simulink model "controladoresDatosProyecto"  (R2022b)
settings: Solver=VariableStepAuto  StartTime=0.0  StopTime=1000  RelTol=1e-3
values from neighbouring files (symbols this model uses):
  kd = k4    (= 0.5686)    [controladoresDatosProyecto.m]
  ki = k1-kp1    (= 2.5726868)    [controladoresDatosProyecto.m]
  kp = k2-kd    (= 54.03607)    [controladoresDatosProyecto.m]
  kp1 = k2    (= 8.2233132)    [controladoresDatosProyecto.m]
  kp2 = k3-kd    (= 0.4314)    [controladoresDatosProyecto.m]
  N = 0.904    [controladoresDatosProyecto.m]
  Tm = 40e-3    (= 0.04)    [controladoresDatosProyecto.m]
undefined symbols (not defined in the file or in its folder): kaw, kpd, kpi
libraries: cstblocks x56
settings Model: Creator=Sebastian  LastModifiedBy=electronica
settings ModelReferenceCC: EnableRefExpFcnMdlSchedulingChecks=on

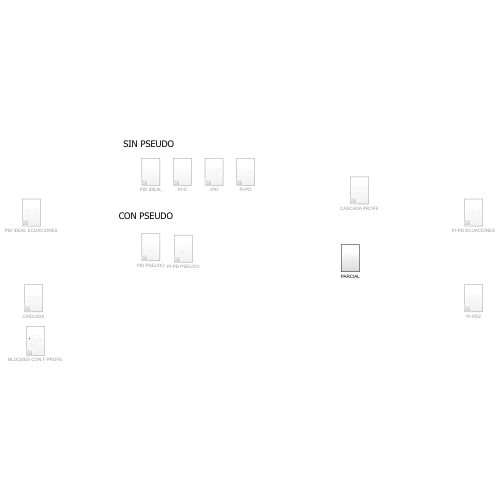
[thumbnail: Simulink's stored preview of the top-level diagram]
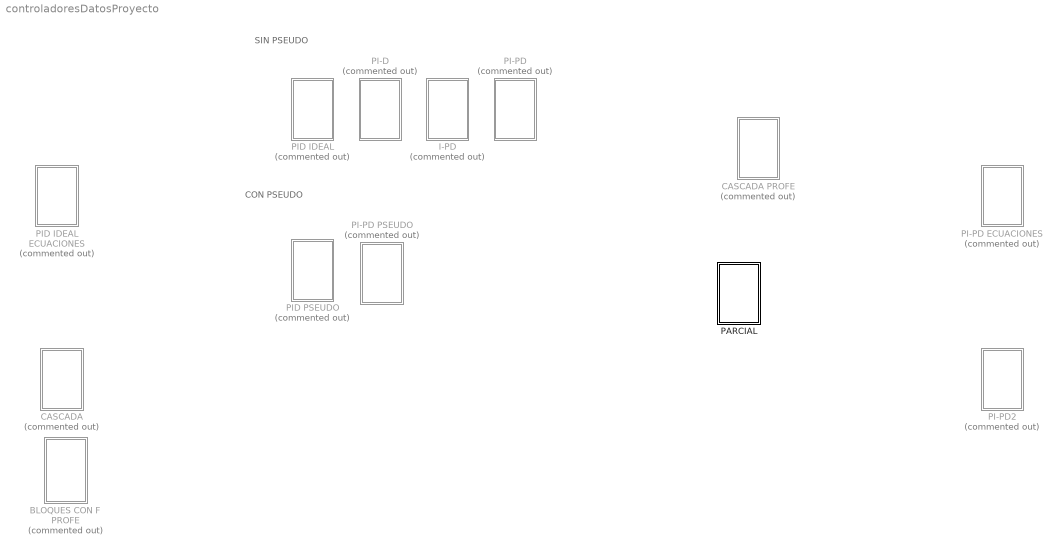
== system controladoresDatosProyecto ==
  note: SIN PSEUDO
  note: CON PSEUDO
  BLOQUES CON F PROFE : Subsystem  Commented=on
  CASCADA : Subsystem  Commented=on
  CASCADA PROFE : Subsystem  Commented=on
  I-PD : Subsystem  Commented=on
  PARCIAL : Subsystem
  PI-D : Subsystem  Commented=on
  PI-PD : Subsystem  Commented=on
  PI-PD ECUACIONES : Subsystem  Commented=on
  PI-PD PSEUDO : Subsystem  Commented=on
  PI-PD2 : Subsystem  Commented=on
  PID IDEAL : Subsystem  Commented=on
  PID IDEAL ECUACIONES : Subsystem  Commented=on
  PID PSEUDO : Subsystem  Commented=on

== system controladoresDatosProyecto/BLOQUES CON F PROFE ==
  LTI System : cstblocks/LTI System  sys=g  IC=[]
  LTI System1 : cstblocks/LTI System  sys=C  IC=[]
  LTI System2 : cstblocks/LTI System  sys=F  IC=[]
  LTI System3 : cstblocks/LTI System  sys=gz  IC=[]
  MATLAB Function : MATLAB Function  TreatAsAtomicUnit=on
  Mux : Mux  Inputs=3
  Mux1 : Mux  Inputs=2
  Scope : Scope  NumInputPorts=2
  Step : Step  Time=0  SampleTime=0
  Subtract : Sum
  Subtract1 : Sum  Inputs=+-
  Unit Delay : UnitDelay  InitialCondition=zeros(6,1)  SampleTime=0.2  HasFrameUpgradeWarning=on
  wires:
  LTI System1/1 -> Subtract/2
  LTI System/1 -> Subtract1/2, Mux/2
  Mux1/1 -> Scope/2
  MATLAB Function/2(Con_out) -> Unit Delay/1
  LTI System3/1 -> Mux/3, MATLAB Function/2(Pv)
  Unit Delay/1 -> MATLAB Function/3(Con_ini)
  Mux/1 -> Scope/1
  LTI System2/1 -> Subtract/1
  Step/1 -> Mux/1, LTI System2/1, MATLAB Function/1(Sp), Subtract1/1
  Subtract/1 -> LTI System/1, Mux1/1
  MATLAB Function/1(u) -> LTI System3/1, Mux1/2
  Subtract1/1 -> LTI System1/1

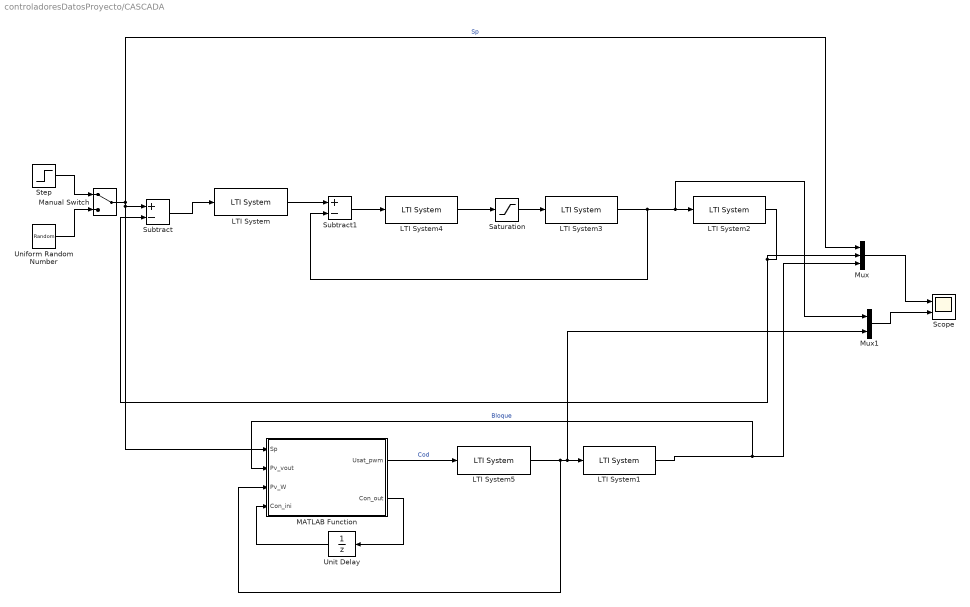
== system controladoresDatosProyecto/CASCADA ==
  LTI System : cstblocks/LTI System  sys=C1  IC=[]
  LTI System1 : cstblocks/LTI System  sys=G1z  IC=[]
  LTI System2 : cstblocks/LTI System  sys=G1z  IC=[]
  LTI System3 : cstblocks/LTI System  sys=G2z  IC=[]
  LTI System4 : cstblocks/LTI System  sys=C2  IC=[]
  LTI System5 : cstblocks/LTI System  sys=G2z  IC=[]
  MATLAB Function : MATLAB Function  TreatAsAtomicUnit=on
  Manual Switch : ManualSwitch
  Mux : Mux  Inputs=3
  Mux1 : Mux  Inputs=2
  Saturation : Saturate  UpperLimit=100  LowerLimit=0
  Scope : Scope  NumInputPorts=2
  Step : Step  Time=5  After=5  SampleTime=5
  Subtract : Sum  Inputs=+-
  Subtract1 : Sum  Inputs=+-
  Uniform Random Number : UniformRandomNumber  Minimum=0  Maximum=5  SampleTime=5
  Unit Delay : UnitDelay  InitialCondition=zeros(8,1)  SampleTime=Tm  HasFrameUpgradeWarning=on
  wires:
  LTI System5/1 -> LTI System1/1, Mux1/2, MATLAB Function/3(Pv_W)
  MATLAB Function/1(Usat_pwm) -> LTI System5/1  "Cod"
  LTI System3/1 -> LTI System2/1, Mux1/1, Subtract1/2
  LTI System4/1 -> Saturation/1
  Subtract1/1 -> LTI System4/1
  Saturation/1 -> LTI System3/1
  LTI System2/1 -> Subtract/2, Mux/2
  Subtract/1 -> LTI System/1
  LTI System/1 -> Subtract1/1
  Mux/1 -> Scope/1
  LTI System1/1 -> Mux/3, MATLAB Function/2(Pv_vout)  "Bloque"
  Step/1 -> Manual Switch/1
  Uniform Random Number/1 -> Manual Switch/2
  Mux1/1 -> Scope/2
  Unit Delay/1 -> MATLAB Function/4(Con_ini)
  Manual Switch/1 -> Mux/1, MATLAB Function/1(Sp), Subtract/1  "Sp"
  MATLAB Function/2(Con_out) -> Unit Delay/1

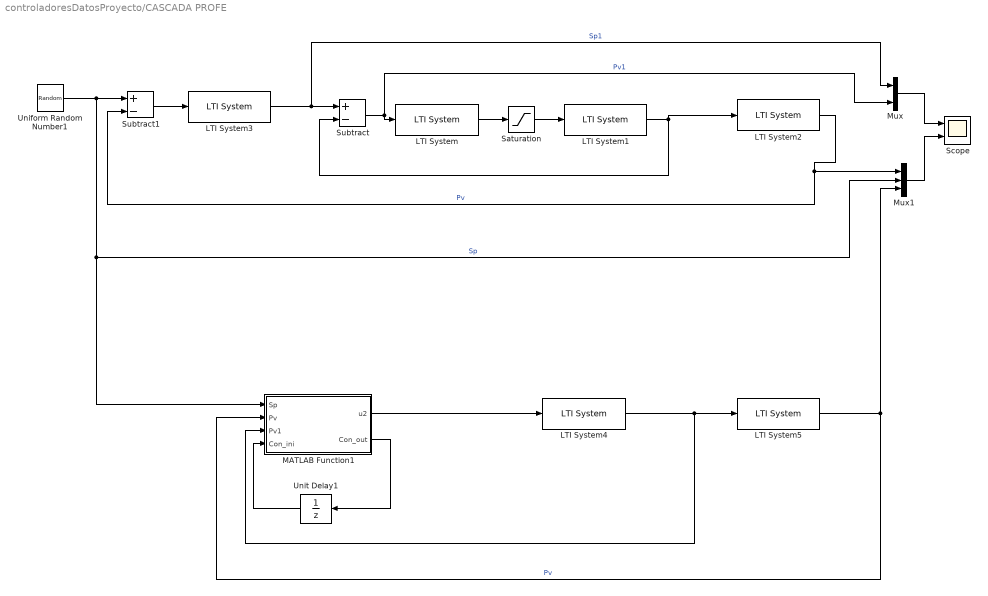
== system controladoresDatosProyecto/CASCADA PROFE ==
  LTI System : cstblocks/LTI System  sys=C1  IC=[]
  LTI System1 : cstblocks/LTI System  sys=G1  IC=[]
  LTI System2 : cstblocks/LTI System  sys=G2  IC=[]
  LTI System3 : cstblocks/LTI System  sys=C2  IC=[]
  LTI System4 : cstblocks/LTI System  sys=g1z  IC=[]
  LTI System5 : cstblocks/LTI System  sys=g2z  IC=[]
  MATLAB Function1 : MATLAB Function  TreatAsAtomicUnit=on
  Mux : Mux  Inputs=2
  Mux1 : Mux  Inputs=3
  Saturation : Saturate  UpperLimit=20  LowerLimit=0
  Scope : Scope  NumInputPorts=2
  Subtract : Sum  Inputs=+-
  Subtract1 : Sum  Inputs=+-
  Uniform Random Number1 : UniformRandomNumber  Minimum=0  Maximum=40  SampleTime=150
  Unit Delay1 : UnitDelay  InitialCondition=zeros(6,1)  SampleTime=Tm  HasFrameUpgradeWarning=on
  wires:
  MATLAB Function1/1(u2) -> LTI System4/1
  MATLAB Function1/2(Con_out) -> Unit Delay1/1
  Unit Delay1/1 -> MATLAB Function1/4(Con_ini)
  LTI System5/1 -> MATLAB Function1/2(Pv), Mux1/3  "Pv"
  LTI System4/1 -> LTI System5/1, MATLAB Function1/3(Pv1)
  LTI System1/1 -> LTI System2/1, Subtract/2
  Subtract/1 -> LTI System/1, Mux/2  "Pv1"
  Subtract1/1 -> LTI System3/1
  Mux/1 -> Scope/1
  LTI System2/1 -> Mux1/1, Subtract1/2  "Pv"
  Mux1/1 -> Scope/2
  Uniform Random Number1/1 -> Subtract1/1, Mux1/2, MATLAB Function1/1(Sp)  "Sp"
  LTI System3/1 -> Subtract/1, Mux/1  "Sp1"
  LTI System/1 -> Saturation/1
  Saturation/1 -> LTI System1/1

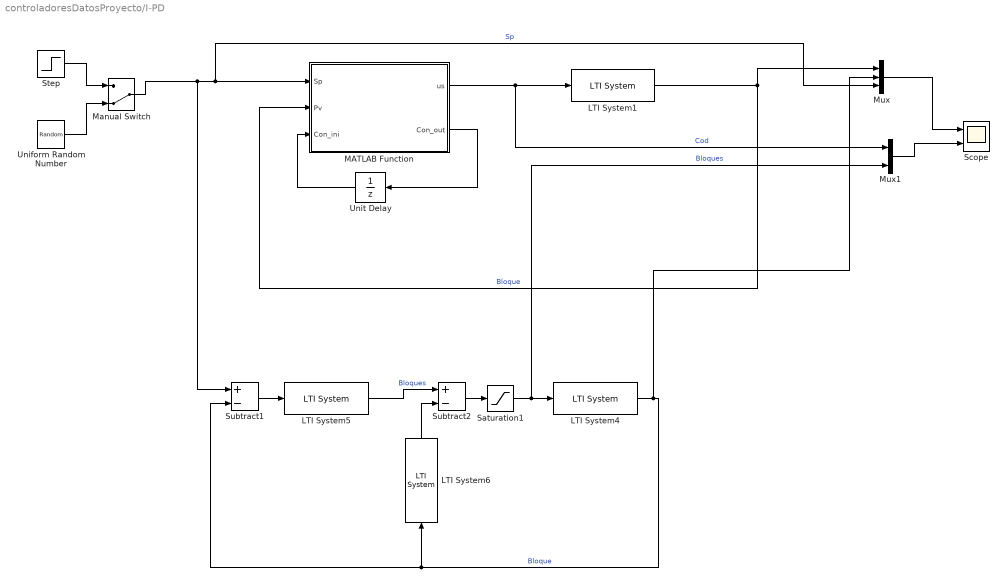
== system controladoresDatosProyecto/I-PD ==
  LTI System1 : cstblocks/LTI System  sys=Gz  IC=[]
  LTI System4 : cstblocks/LTI System  sys=Gz  IC=[]
  LTI System5 : cstblocks/LTI System  sys=Ci  IC=[]
  LTI System6 : cstblocks/LTI System  sys=Cpd  IC=[]
  MATLAB Function : MATLAB Function  TreatAsAtomicUnit=on
  Manual Switch : ManualSwitch  CurrentSetting=0
  Mux : Mux  Inputs=3
  Mux1 : Mux  Inputs=2
  Saturation1 : Saturate  UpperLimit=100  LowerLimit=0
  Scope : Scope  NumInputPorts=2
  Step : Step  Time=100  Before=18  After=15  SampleTime=0
  Subtract1 : Sum  Inputs=+-
  Subtract2 : Sum  Inputs=+-
  Uniform Random Number : UniformRandomNumber  Minimum=0  Maximum=5  SampleTime=5
  Unit Delay : UnitDelay  InitialCondition=zeros(3,1)  SampleTime=Tm  HasFrameUpgradeWarning=on
  wires:
  MATLAB Function/2(Con_out) -> Unit Delay/1
  Unit Delay/1 -> MATLAB Function/3(Con_ini)
  Mux1/1 -> Scope/2
  Uniform Random Number/1 -> Manual Switch/2
  Step/1 -> Manual Switch/1
  MATLAB Function/1(us) -> Mux1/1, LTI System1/1  "Cod"
  LTI System1/1 -> Mux/1, MATLAB Function/2(Pv)  "Bloque"
  Mux/1 -> Scope/1
  Subtract2/1 -> Saturation1/1
  Saturation1/1 -> Mux1/2, LTI System4/1  "Bloques"
  LTI System4/1 -> Mux/2, LTI System6/1, Subtract1/2  "Bloque"
  Manual Switch/1 -> Subtract1/1, Mux/3, MATLAB Function/1(Sp)  "Sp"
  LTI System6/1 -> Subtract2/2
  LTI System5/1 -> Subtract2/1  "Bloques"
  Subtract1/1 -> LTI System5/1

== system controladoresDatosProyecto/PARCIAL ==
  CASCADA : cstblocks/LTI System  sys=g2z  IC=[]
  LTI System8 : cstblocks/LTI System  sys=g1z  IC=[]
  Mux2 : Mux  Inputs=3
  Mux3 : Mux  Inputs=2
  PI-D : cstblocks/LTI System  sys=gz  IC=[]
  SETPOINT : UniformRandomNumber  Minimum=0  Maximum=40  SampleTime=70
  Scope1 : Scope  NumInputPorts=2
  UCASCADA : MATLAB Function  TreatAsAtomicUnit=on
  UPI-D : MATLAB Function  TreatAsAtomicUnit=on
  Unit Delay1 : UnitDelay  InitialCondition=zeros(2,1)  SampleTime=Tm  HasFrameUpgradeWarning=on
  Unit Delay2 : UnitDelay  InitialCondition=zeros(6,1)  SampleTime=Tm  HasFrameUpgradeWarning=on
  wires:
  PI-D/1 -> Mux2/2, UPI-D/2(Pv)
  Mux3/1 -> Scope1/2
  UPI-D/1(us) -> Mux3/1, PI-D/1
  Unit Delay1/1 -> UPI-D/3(Con_ini)
  UPI-D/2(Con_out) -> Unit Delay1/1
  SETPOINT/1 -> Mux2/1, UPI-D/1(Sp), UCASCADA/1(Sp)
  Mux2/1 -> Scope1/1
  UCASCADA/2(Con_out) -> Unit Delay2/1
  LTI System8/1 -> CASCADA/1, UCASCADA/3(Pv1)
  UCASCADA/1(u2) -> Mux3/2, LTI System8/1
  Unit Delay2/1 -> UCASCADA/4(Con_ini)
  CASCADA/1 -> Mux2/3, UCASCADA/2(Pv)

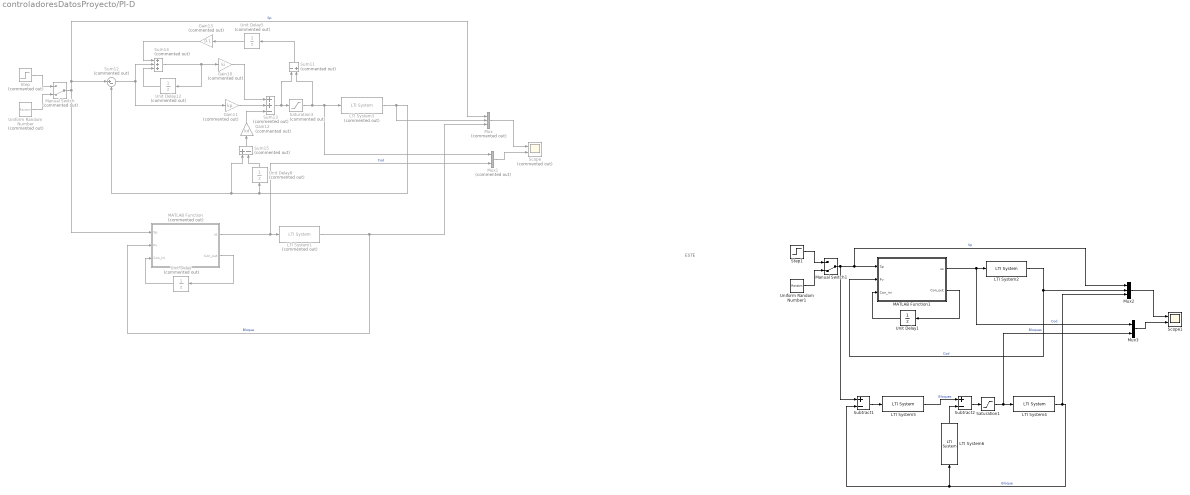
== system controladoresDatosProyecto/PI-D ==
  note: ESTE
  Gain10 : Gain  Commented=on  Gain=ki
  Gain11 : Gain  Commented=on  Gain=kp
  Gain12 : Gain  Commented=on  Gain=kd
  Gain13 : Gain  Commented=on  Gain=0.1
  LTI System1 : cstblocks/LTI System  Commented=on  sys=G1z  IC=[]
  LTI System2 : cstblocks/LTI System  sys=Gz  IC=[]
  LTI System3 : cstblocks/LTI System  Commented=on  sys=G1z  IC=[]
  LTI System4 : cstblocks/LTI System  sys=Gz  IC=[]
  LTI System5 : cstblocks/LTI System  sys=Cpi  IC=[]
  LTI System6 : cstblocks/LTI System  sys=Cd  IC=[]
  MATLAB Function : MATLAB Function  Commented=on  TreatAsAtomicUnit=on
  MATLAB Function1 : MATLAB Function  TreatAsAtomicUnit=on
  Manual Switch : ManualSwitch  Commented=on  CurrentSetting=0
  Manual Switch1 : ManualSwitch  CurrentSetting=0
  Mux : Mux  Commented=on  Inputs=3
  Mux1 : Mux  Commented=on  Inputs=2
  Mux2 : Mux  Inputs=3
  Mux3 : Mux  Inputs=2
  Saturation1 : Saturate  UpperLimit=100  LowerLimit=0
  Saturation3 : Saturate  Commented=on  UpperLimit=100  LowerLimit=0
  Scope : Scope  Commented=on  NumInputPorts=2
  Scope1 : Scope  NumInputPorts=2
  Step : Step  Commented=on  Time=100  Before=18  After=15  SampleTime=0
  Step1 : Step  Time=100  Before=18  After=15  SampleTime=0
  Subtract1 : Sum  Inputs=+-
  Subtract2 : Sum  Inputs=+-
  Sum11 : Sum  Commented=on  Inputs=-+
  Sum12 : Sum  Commented=on  Inputs=|+-
  Sum13 : Sum  Commented=on  Inputs=++-
  Sum14 : Sum  Commented=on  Inputs=+++
  Sum15 : Sum  Commented=on  Inputs=+-
  Uniform Random Number : UniformRandomNumber  Commented=on  Minimum=0  Maximum=5  SampleTime=5
  Uniform Random Number1 : UniformRandomNumber  Minimum=0  Maximum=4.5  SampleTime=10
  Unit Delay : UnitDelay  Commented=on  InitialCondition=zeros(3,1)  SampleTime=Tm  HasFrameUpgradeWarning=on
  Unit Delay1 : UnitDelay  InitialCondition=zeros(3,1)  SampleTime=Tm  HasFrameUpgradeWarning=on
  Unit Delay12 : UnitDelay  Commented=on  SampleTime=Tm  HasFrameUpgradeWarning=on
  Unit Delay5 : UnitDelay  Commented=on  SampleTime=Tm  HasFrameUpgradeWarning=on
  Unit Delay8 : UnitDelay  Commented=on  SampleTime=Tm  HasFrameUpgradeWarning=on
  wires:
  Mux/1 -> Scope/1
  LTI System1/1 -> MATLAB Function/2(Pv), Mux/3  "Bloque"
  MATLAB Function/1(us) -> Mux1/2, LTI System1/1  "Cod"
  Step/1 -> Manual Switch/1
  Uniform Random Number/1 -> Manual Switch/2
  Mux1/1 -> Scope/2
  Unit Delay/1 -> MATLAB Function/3(Con_ini)
  Manual Switch/1 -> Sum12/1, Mux/1, MATLAB Function/1(Sp)  "Sp"
  MATLAB Function/2(Con_out) -> Unit Delay/1
  Sum15/1 -> Gain12/1
  Gain13/1 -> Sum14/1
  Saturation3/1 -> Sum11/2, Mux1/1, LTI System3/1
  LTI System3/1 -> Mux/2, Unit Delay8/1, Sum12/2, Sum15/1
  Sum14/1 -> Gain10/1, Unit Delay12/1
  Gain10/1 -> Sum13/1
  Unit Delay8/1 -> Sum15/2
  Gain11/1 -> Sum13/2
  Unit Delay5/1 -> Gain13/1
  Unit Delay12/1 -> Sum14/3
  Gain12/1 -> Sum13/3
  Sum11/1 -> Unit Delay5/1
  Sum13/1 -> Saturation3/1, Sum11/1
  Sum12/1 -> Sum14/2, Gain11/1
  Step1/1 -> Manual Switch1/1
  Manual Switch1/1 -> Subtract1/1, Mux2/1, MATLAB Function1/1(Sp)  "Sp"
  Subtract1/1 -> LTI System5/1
  Unit Delay1/1 -> MATLAB Function1/3(Con_ini)
  LTI System4/1 -> Mux2/3, LTI System6/1, Subtract1/2  "Bloque"
  Mux2/1 -> Scope1/1
  Mux3/1 -> Scope1/2
  LTI System6/1 -> Subtract2/2
  Saturation1/1 -> Mux3/2, LTI System4/1  "Bloques"
  MATLAB Function1/1(us) -> Mux3/1, LTI System2/1  "Cod"
  Subtract2/1 -> Saturation1/1
  LTI System2/1 -> Mux2/2, MATLAB Function1/2(Pv)  "Cod"
  LTI System5/1 -> Subtract2/1  "Bloques"
  MATLAB Function1/2(Con_out) -> Unit Delay1/1
  Uniform Random Number1/1 -> Manual Switch1/2

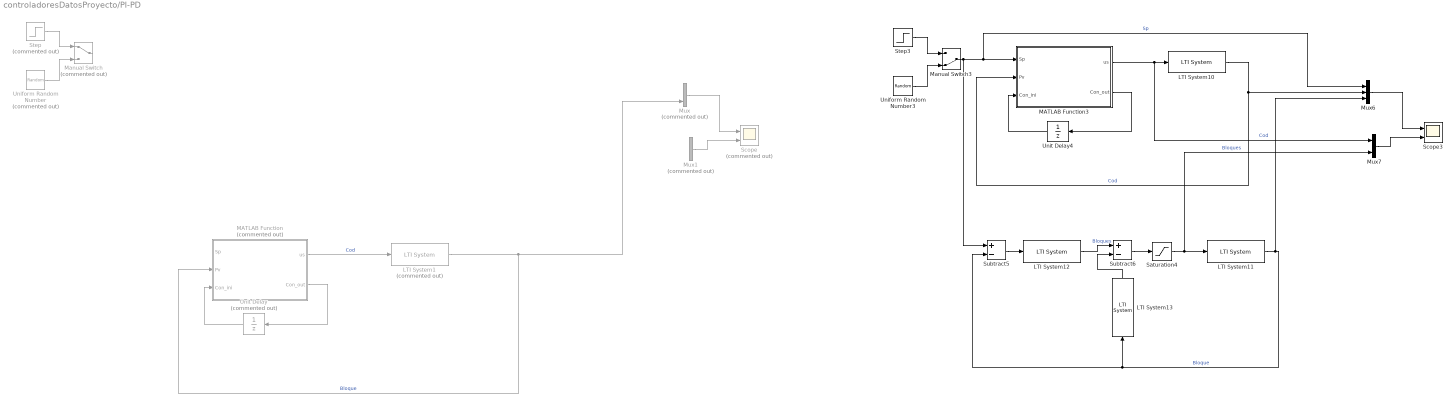
== system controladoresDatosProyecto/PI-PD ==
  LTI System1 : cstblocks/LTI System  Commented=on  sys=G1z  IC=[]
  LTI System10 : cstblocks/LTI System  sys=Gz  IC=[]
  LTI System11 : cstblocks/LTI System  sys=Gz  IC=[]
  LTI System12 : cstblocks/LTI System  sys=Cpi  IC=[]
  LTI System13 : cstblocks/LTI System  sys=Cpd  IC=[]
  MATLAB Function : MATLAB Function  Commented=on  TreatAsAtomicUnit=on
  MATLAB Function3 : MATLAB Function  TreatAsAtomicUnit=on
  Manual Switch : ManualSwitch  Commented=on
  Manual Switch3 : ManualSwitch  CurrentSetting=0
  Mux : Mux  Commented=on  Inputs=3
  Mux1 : Mux  Commented=on  Inputs=2
  Mux6 : Mux  Inputs=3
  Mux7 : Mux  Inputs=2
  Saturation4 : Saturate  UpperLimit=100  LowerLimit=0
  Scope : Scope  Commented=on  NumInputPorts=2
  Scope3 : Scope  NumInputPorts=2
  Step : Step  Commented=on  Time=5  After=3  SampleTime=5
  Step3 : Step  Time=0  After=20  SampleTime=0
  Subtract5 : Sum  Inputs=+-
  Subtract6 : Sum  Inputs=+-
  Uniform Random Number : UniformRandomNumber  Commented=on  Minimum=0  Maximum=5  SampleTime=5
  Uniform Random Number3 : UniformRandomNumber  Minimum=0  Maximum=4.5  SampleTime=10
  Unit Delay : UnitDelay  Commented=on  InitialCondition=zeros(3,1)  SampleTime=Tm  HasFrameUpgradeWarning=on
  Unit Delay4 : UnitDelay  InitialCondition=zeros(3,1)  SampleTime=Tm  HasFrameUpgradeWarning=on
  wires:
  Mux/1 -> Scope/1
  LTI System1/1 -> MATLAB Function/2(Pv), Mux/3  "Bloque"
  MATLAB Function/1(us) -> LTI System1/1  "Cod"
  Step/1 -> Manual Switch/1
  Uniform Random Number/1 -> Manual Switch/2
  Mux1/1 -> Scope/2
  Unit Delay/1 -> MATLAB Function/3(Con_ini)
  MATLAB Function/2(Con_out) -> Unit Delay/1
  MATLAB Function3/1(us) -> Mux7/1, LTI System10/1  "Cod"
  LTI System10/1 -> Mux6/2, MATLAB Function3/2(Pv)  "Cod"
  Unit Delay4/1 -> MATLAB Function3/3(Con_ini)
  LTI System11/1 -> Mux6/3, LTI System13/1, Subtract5/2  "Bloque"
  Mux6/1 -> Scope3/1
  Saturation4/1 -> Mux7/2, LTI System11/1  "Bloques"
  Step3/1 -> Manual Switch3/1
  Subtract6/1 -> Saturation4/1
  LTI System12/1 -> Subtract6/1  "Bloques"
  Mux7/1 -> Scope3/2
  LTI System13/1 -> Subtract6/2
  Manual Switch3/1 -> Subtract5/1, Mux6/1, MATLAB Function3/1(Sp)  "Sp"
  Subtract5/1 -> LTI System12/1
  MATLAB Function3/2(Con_out) -> Unit Delay4/1
  Uniform Random Number3/1 -> Manual Switch3/2

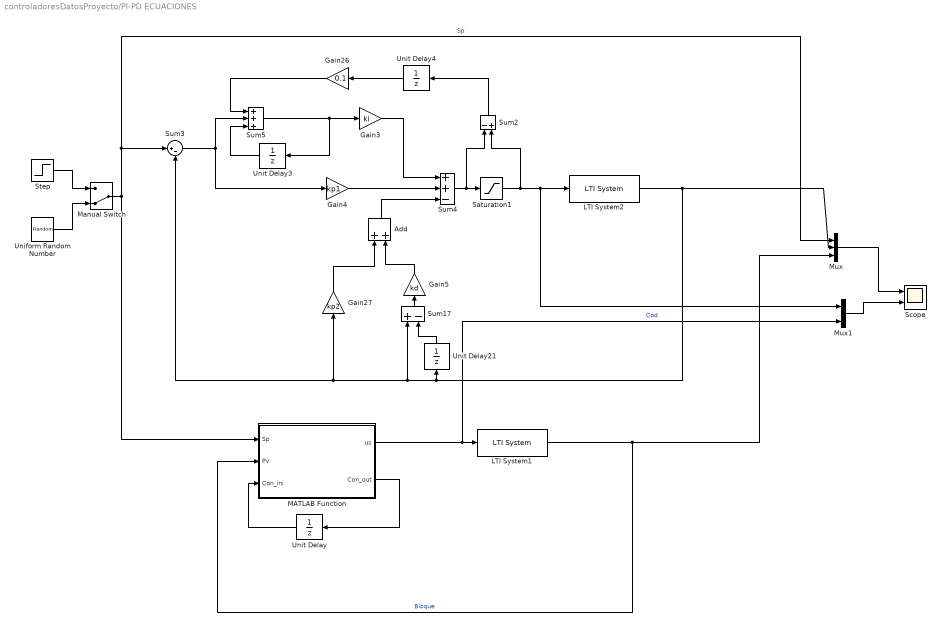
== system controladoresDatosProyecto/PI-PD ECUACIONES ==
  Add : Sum
  Gain26 : Gain  Gain=0.1
  Gain27 : Gain  Gain=kp2
  Gain3 : Gain  Gain=ki
  Gain4 : Gain  Gain=kp1
  Gain5 : Gain  Gain=kd
  LTI System1 : cstblocks/LTI System  sys=G1z  IC=[]
  LTI System2 : cstblocks/LTI System  sys=G1z  IC=[]
  MATLAB Function : MATLAB Function  TreatAsAtomicUnit=on
  Manual Switch : ManualSwitch  CurrentSetting=0
  Mux : Mux  Inputs=3
  Mux1 : Mux  Inputs=2
  Saturation1 : Saturate  UpperLimit=100  LowerLimit=0
  Scope : Scope  NumInputPorts=2
  Step : Step  Time=5  After=3  SampleTime=5
  Sum17 : Sum  Inputs=+-
  Sum2 : Sum  Inputs=-+
  Sum3 : Sum  Inputs=|+-
  Sum4 : Sum  Inputs=++-
  Sum5 : Sum  Inputs=+++
  Uniform Random Number : UniformRandomNumber  Minimum=0  Maximum=5  SampleTime=5
  Unit Delay : UnitDelay  InitialCondition=zeros(4,1)  SampleTime=Tm  HasFrameUpgradeWarning=on
  Unit Delay21 : UnitDelay  SampleTime=Tm  HasFrameUpgradeWarning=on
  Unit Delay3 : UnitDelay  SampleTime=Tm  HasFrameUpgradeWarning=on
  Unit Delay4 : UnitDelay  SampleTime=Tm  HasFrameUpgradeWarning=on
  wires:
  LTI System2/1 -> Sum17/1, Sum3/2, Gain27/1, Unit Delay21/1, Mux/2
  Gain26/1 -> Sum5/1
  Unit Delay21/1 -> Sum17/2
  Gain3/1 -> Sum4/1
  Unit Delay4/1 -> Gain26/1
  Sum5/1 -> Unit Delay3/1, Gain3/1
  Unit Delay3/1 -> Sum5/3
  Sum4/1 -> Sum2/1, Saturation1/1
  Saturation1/1 -> LTI System2/1, Mux1/1, Sum2/2
  Gain4/1 -> Sum4/2
  Sum3/1 -> Gain4/1, Sum5/2
  Gain27/1 -> Add/1
  Sum17/1 -> Gain5/1
  Gain5/1 -> Add/2
  Add/1 -> Sum4/3
  Sum2/1 -> Unit Delay4/1
  MATLAB Function/2(Con_out) -> Unit Delay/1
  Manual Switch/1 -> MATLAB Function/1(Sp), Mux/1, Sum3/1  "Sp"
  Unit Delay/1 -> MATLAB Function/3(Con_ini)
  Mux1/1 -> Scope/2
  Uniform Random Number/1 -> Manual Switch/2
  Step/1 -> Manual Switch/1
  MATLAB Function/1(us) -> LTI System1/1, Mux1/2  "Cod"
  LTI System1/1 -> Mux/3, MATLAB Function/2(Pv)  "Bloque"
  Mux/1 -> Scope/1

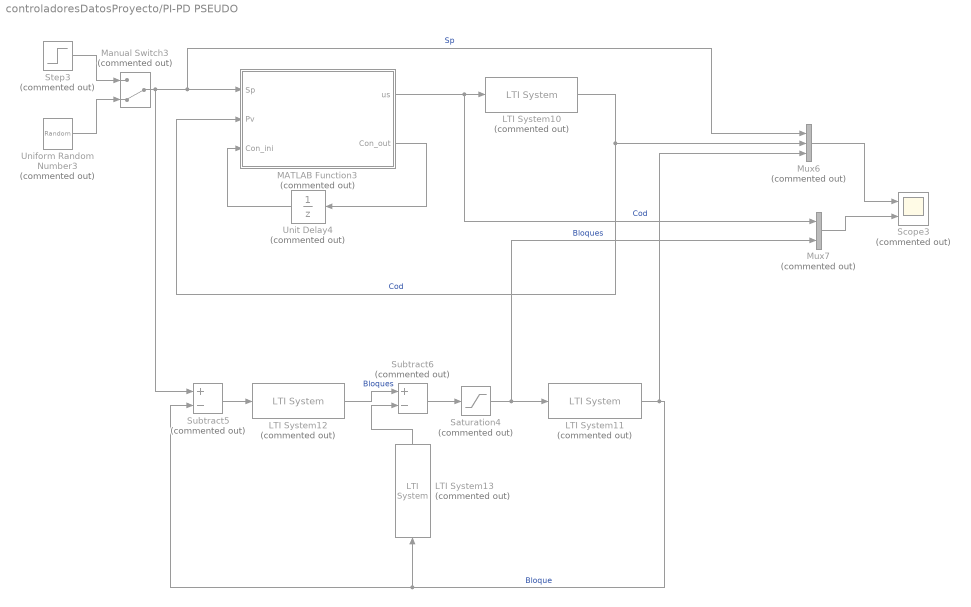
== system controladoresDatosProyecto/PI-PD PSEUDO ==
  LTI System10 : cstblocks/LTI System  Commented=on  sys=Gz  IC=[]
  LTI System11 : cstblocks/LTI System  Commented=on  sys=Gz  IC=[]
  LTI System12 : cstblocks/LTI System  Commented=on  sys=Cpi  IC=[]
  LTI System13 : cstblocks/LTI System  Commented=on  sys=Cpds  IC=[]
  MATLAB Function3 : MATLAB Function  Commented=on  TreatAsAtomicUnit=on
  Manual Switch3 : ManualSwitch  Commented=on  CurrentSetting=0
  Mux6 : Mux  Commented=on  Inputs=3
  Mux7 : Mux  Commented=on  Inputs=2
  Saturation4 : Saturate  Commented=on  UpperLimit=100  LowerLimit=0
  Scope3 : Scope  Commented=on  NumInputPorts=2
  Step3 : Step  Commented=on  Time=0  After=20  SampleTime=0
  Subtract5 : Sum  Commented=on  Inputs=+-
  Subtract6 : Sum  Commented=on  Inputs=+-
  Uniform Random Number3 : UniformRandomNumber  Commented=on  Minimum=0  Maximum=4.5  SampleTime=5
  Unit Delay4 : UnitDelay  Commented=on  InitialCondition=zeros(4,1)  SampleTime=Tm  HasFrameUpgradeWarning=on
  wires:
  Mux7/1 -> Scope3/2
  Manual Switch3/1 -> Subtract5/1, Mux6/1, MATLAB Function3/1(Sp)  "Sp"
  Saturation4/1 -> Mux7/2, LTI System11/1  "Bloques"
  LTI System10/1 -> Mux6/2, MATLAB Function3/2(Pv)  "Cod"
  Step3/1 -> Manual Switch3/1
  LTI System12/1 -> Subtract6/1  "Bloques"
  Subtract6/1 -> Saturation4/1
  LTI System11/1 -> Mux6/3, LTI System13/1, Subtract5/2  "Bloque"
  LTI System13/1 -> Subtract6/2
  Unit Delay4/1 -> MATLAB Function3/3(Con_ini)
  Mux6/1 -> Scope3/1
  MATLAB Function3/1(us) -> Mux7/1, LTI System10/1  "Cod"
  Subtract5/1 -> LTI System12/1
  MATLAB Function3/2(Con_out) -> Unit Delay4/1
  Uniform Random Number3/1 -> Manual Switch3/2

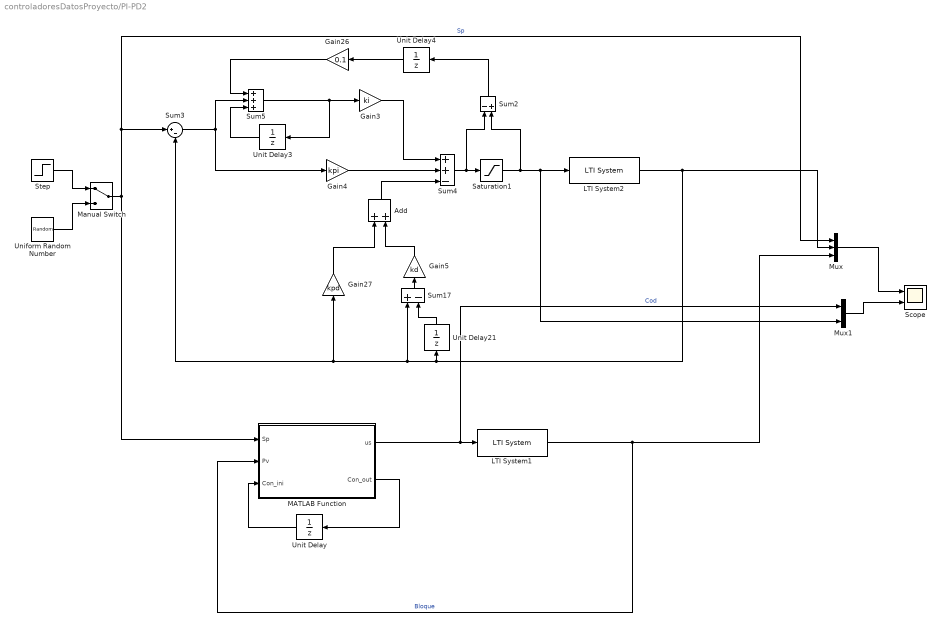
== system controladoresDatosProyecto/PI-PD2 ==
  Add : Sum
  Gain26 : Gain  Gain=0.1
  Gain27 : Gain  Gain=kpd
  Gain3 : Gain  Gain=ki
  Gain4 : Gain  Gain=kpi
  Gain5 : Gain  Gain=kd
  LTI System1 : cstblocks/LTI System  sys=Gz  IC=[]
  LTI System2 : cstblocks/LTI System  sys=Gz  IC=[]
  MATLAB Function : MATLAB Function  TreatAsAtomicUnit=on
  Manual Switch : ManualSwitch
  Mux : Mux  Inputs=3
  Mux1 : Mux  Inputs=2
  Saturation1 : Saturate  UpperLimit=100  LowerLimit=0
  Scope : Scope  NumInputPorts=2
  Step : Step  Time=5  After=20  SampleTime=5
  Sum17 : Sum  Inputs=+-
  Sum2 : Sum  Inputs=-+
  Sum3 : Sum  Inputs=|+-
  Sum4 : Sum  Inputs=++-
  Sum5 : Sum  Inputs=+++
  Uniform Random Number : UniformRandomNumber  Minimum=0  Maximum=5  SampleTime=5
  Unit Delay : UnitDelay  InitialCondition=zeros(4,1)  SampleTime=Tm  HasFrameUpgradeWarning=on
  Unit Delay21 : UnitDelay  SampleTime=Tm  HasFrameUpgradeWarning=on
  Unit Delay3 : UnitDelay  SampleTime=Tm  HasFrameUpgradeWarning=on
  Unit Delay4 : UnitDelay  SampleTime=Tm  HasFrameUpgradeWarning=on
  wires:
  Mux/1 -> Scope/1
  LTI System1/1 -> MATLAB Function/2(Pv), Mux/3  "Bloque"
  MATLAB Function/1(us) -> LTI System1/1, Mux1/1  "Cod"
  Step/1 -> Manual Switch/1
  Uniform Random Number/1 -> Manual Switch/2
  Mux1/1 -> Scope/2
  Unit Delay/1 -> MATLAB Function/3(Con_ini)
  Manual Switch/1 -> Sum3/1, Mux/1, MATLAB Function/1(Sp)  "Sp"
  MATLAB Function/2(Con_out) -> Unit Delay/1
  Sum3/1 -> Sum5/2, Gain4/1
  Sum4/1 -> Saturation1/1, Sum2/1
  Gain5/1 -> Add/2
  Add/1 -> Sum4/3
  Unit Delay21/1 -> Sum17/2
  Gain27/1 -> Add/1
  LTI System2/1 -> Mux/2, Unit Delay21/1, Gain27/1, Sum3/2, Sum17/1
  Saturation1/1 -> Sum2/2, Mux1/2, LTI System2/1
  Gain26/1 -> Sum5/1
  Gain4/1 -> Sum4/2
  Unit Delay4/1 -> Gain26/1
  Gain3/1 -> Sum4/1
  Sum5/1 -> Gain3/1, Unit Delay3/1
  Sum17/1 -> Gain5/1
  Unit Delay3/1 -> Sum5/3
  Sum2/1 -> Unit Delay4/1

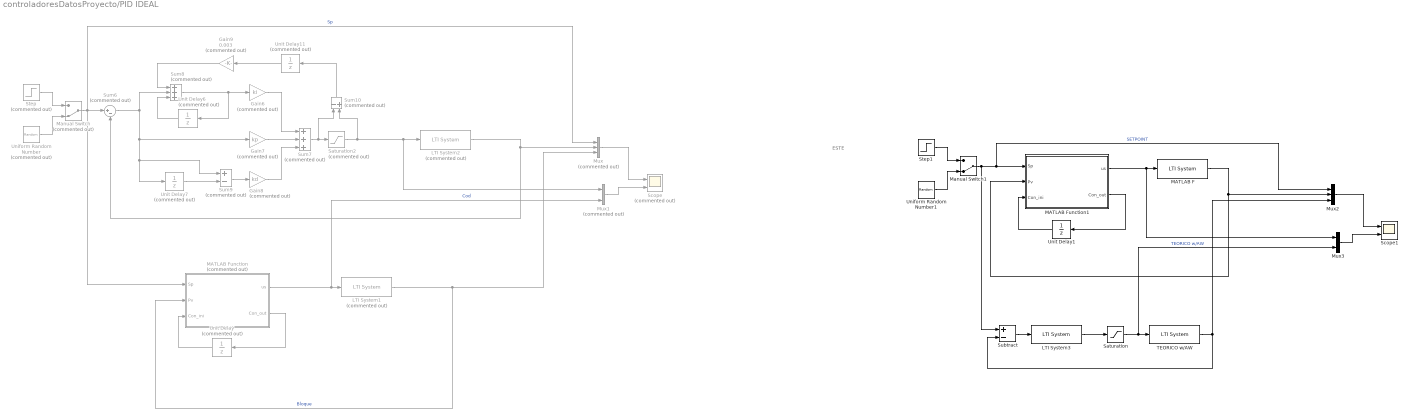
== system controladoresDatosProyecto/PID IDEAL ==
  note: ESTE
  Gain6 : Gain  Commented=on  Gain=ki
  Gain7 : Gain  Commented=on  Gain=kp
  Gain8 : Gain  Commented=on  Gain=kd
  Gain9 : Gain  Commented=on  Gain=0.003
  LTI System1 : cstblocks/LTI System  Commented=on  sys=G1z  IC=[]
  LTI System2 : cstblocks/LTI System  Commented=on  sys=G1z  IC=[]
  LTI System3 : cstblocks/LTI System  sys=Cpid  IC=[]
  MATLAB F : cstblocks/LTI System  sys=Gz  IC=[]
  MATLAB Function : MATLAB Function  Commented=on  TreatAsAtomicUnit=on
  MATLAB Function1 : MATLAB Function  TreatAsAtomicUnit=on
  Manual Switch : ManualSwitch  Commented=on  CurrentSetting=0
  Manual Switch1 : ManualSwitch  CurrentSetting=0
  Mux : Mux  Commented=on  Inputs=3
  Mux1 : Mux  Commented=on  Inputs=2
  Mux2 : Mux  Inputs=3
  Mux3 : Mux  Inputs=2
  Saturation : Saturate  UpperLimit=100  LowerLimit=0
  Saturation2 : Saturate  Commented=on  UpperLimit=100  LowerLimit=0
  Scope : Scope  Commented=on  NumInputPorts=2
  Scope1 : Scope  NumInputPorts=2
  Step : Step  Commented=on  Time=100  Before=18  After=15  SampleTime=0
  Step1 : Step  Time=100  Before=18  After=15  SampleTime=0
  Subtract : Sum  Inputs=+-
  Sum10 : Sum  Commented=on  Inputs=-+
  Sum6 : Sum  Commented=on  Inputs=|+-
  Sum7 : Sum  Commented=on  Inputs=+++
  Sum8 : Sum  Commented=on  Inputs=+++
  Sum9 : Sum  Commented=on  Inputs=+-
  TEORICO w/AW : cstblocks/LTI System  sys=Gz  IC=[]
  Uniform Random Number : UniformRandomNumber  Commented=on  Minimum=0  Maximum=5  SampleTime=5
  Uniform Random Number1 : UniformRandomNumber  Minimum=0  Maximum=4.5  SampleTime=10
  Unit Delay : UnitDelay  Commented=on  InitialCondition=zeros(3,1)  SampleTime=Tm  HasFrameUpgradeWarning=on
  Unit Delay1 : UnitDelay  InitialCondition=zeros(3,1)  SampleTime=Tm  HasFrameUpgradeWarning=on
  Unit Delay11 : UnitDelay  Commented=on  SampleTime=Tm  HasFrameUpgradeWarning=on
  Unit Delay6 : UnitDelay  Commented=on  SampleTime=Tm  HasFrameUpgradeWarning=on
  Unit Delay7 : UnitDelay  Commented=on  SampleTime=Tm  HasFrameUpgradeWarning=on
  wires:
  Sum8/1 -> Gain6/1, Unit Delay6/1
  Saturation2/1 -> Sum10/2, Mux1/1, LTI System2/1
  Sum7/1 -> Saturation2/1, Sum10/1
  Mux/1 -> Scope/1
  LTI System1/1 -> MATLAB Function/2(Pv), Mux/3  "Bloque"
  Sum6/1 -> Sum8/2, Gain7/1, Unit Delay7/1, Sum9/1
  MATLAB Function/1(us) -> Mux1/2, LTI System1/1  "Cod"
  Sum9/1 -> Gain8/1
  Step/1 -> Manual Switch/1
  Unit Delay7/1 -> Sum9/2
  Gain8/1 -> Sum7/3
  Gain6/1 -> Sum7/1
  Gain9/1 -> Sum8/1
  Uniform Random Number/1 -> Manual Switch/2
  Mux1/1 -> Scope/2
  Unit Delay/1 -> MATLAB Function/3(Con_ini)
  Manual Switch/1 -> MATLAB Function/1(Sp), Mux/1, Sum6/1  "Sp"
  LTI System2/1 -> Mux/2, Sum6/2
  Unit Delay6/1 -> Sum8/3
  Unit Delay11/1 -> Gain9/1
  Sum10/1 -> Unit Delay11/1
  MATLAB Function/2(Con_out) -> Unit Delay/1
  Gain7/1 -> Sum7/2
  Manual Switch1/1 -> Subtract/1, Mux2/1, MATLAB Function1/1(Sp)  "SETPOINT"
  Mux2/1 -> Scope1/1
  Uniform Random Number1/1 -> Manual Switch1/2
  MATLAB Function1/2(Con_out) -> Unit Delay1/1
  Subtract/1 -> LTI System3/1
  TEORICO w/AW/1 -> Mux2/3, Subtract/2
  MATLAB Function1/1(us) -> Mux3/1, MATLAB F/1
  Unit Delay1/1 -> MATLAB Function1/3(Con_ini)
  MATLAB F/1 -> MATLAB Function1/2(Pv), Mux2/2
  Saturation/1 -> Mux3/2, TEORICO w/AW/1  "TEORICO w/AW"
  Step1/1 -> Manual Switch1/1
  Mux3/1 -> Scope1/2
  LTI System3/1 -> Saturation/1

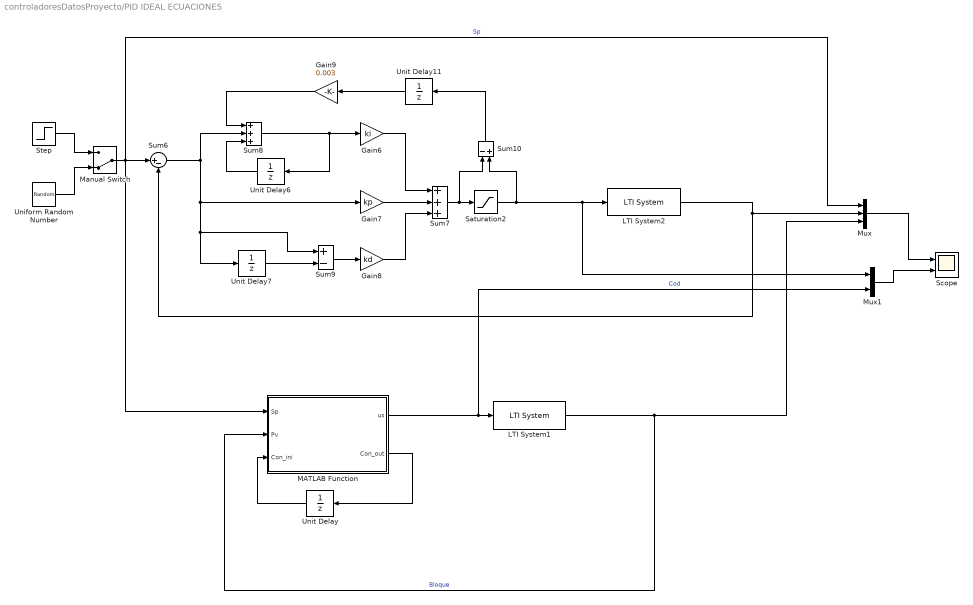
== system controladoresDatosProyecto/PID IDEAL ECUACIONES ==
  Gain6 : Gain  Gain=ki
  Gain7 : Gain  Gain=kp
  Gain8 : Gain  Gain=kd
  Gain9 : Gain  Gain=0.003
  LTI System1 : cstblocks/LTI System  sys=G1z  IC=[]
  LTI System2 : cstblocks/LTI System  sys=G1z  IC=[]
  MATLAB Function : MATLAB Function  TreatAsAtomicUnit=on
  Manual Switch : ManualSwitch  CurrentSetting=0
  Mux : Mux  Inputs=3
  Mux1 : Mux  Inputs=2
  Saturation2 : Saturate  UpperLimit=100  LowerLimit=0
  Scope : Scope  NumInputPorts=2
  Step : Step  Time=100  Before=18  After=15  SampleTime=0
  Sum10 : Sum  Inputs=-+
  Sum6 : Sum  Inputs=|+-
  Sum7 : Sum  Inputs=+++
  Sum8 : Sum  Inputs=+++
  Sum9 : Sum  Inputs=+-
  Uniform Random Number : UniformRandomNumber  Minimum=0  Maximum=5  SampleTime=5
  Unit Delay : UnitDelay  InitialCondition=zeros(4,1)  SampleTime=Tm  HasFrameUpgradeWarning=on
  Unit Delay11 : UnitDelay  SampleTime=Tm  HasFrameUpgradeWarning=on
  Unit Delay6 : UnitDelay  SampleTime=Tm  HasFrameUpgradeWarning=on
  Unit Delay7 : UnitDelay  SampleTime=Tm  HasFrameUpgradeWarning=on
  wires:
  Gain7/1 -> Sum7/2
  MATLAB Function/2(Con_out) -> Unit Delay/1
  Sum10/1 -> Unit Delay11/1
  Unit Delay11/1 -> Gain9/1
  Unit Delay6/1 -> Sum8/3
  LTI System2/1 -> Sum6/2, Mux/2
  Manual Switch/1 -> Sum6/1, Mux/1, MATLAB Function/1(Sp)  "Sp"
  Unit Delay/1 -> MATLAB Function/3(Con_ini)
  Mux1/1 -> Scope/2
  Uniform Random Number/1 -> Manual Switch/2
  Gain9/1 -> Sum8/1
  Gain6/1 -> Sum7/1
  Gain8/1 -> Sum7/3
  Unit Delay7/1 -> Sum9/2
  Step/1 -> Manual Switch/1
  Sum9/1 -> Gain8/1
  MATLAB Function/1(us) -> LTI System1/1, Mux1/2  "Cod"
  Sum6/1 -> Sum9/1, Unit Delay7/1, Gain7/1, Sum8/2
  LTI System1/1 -> Mux/3, MATLAB Function/2(Pv)  "Bloque"
  Mux/1 -> Scope/1
  Sum7/1 -> Sum10/1, Saturation2/1
  Saturation2/1 -> LTI System2/1, Mux1/1, Sum10/2
  Sum8/1 -> Unit Delay6/1, Gain6/1

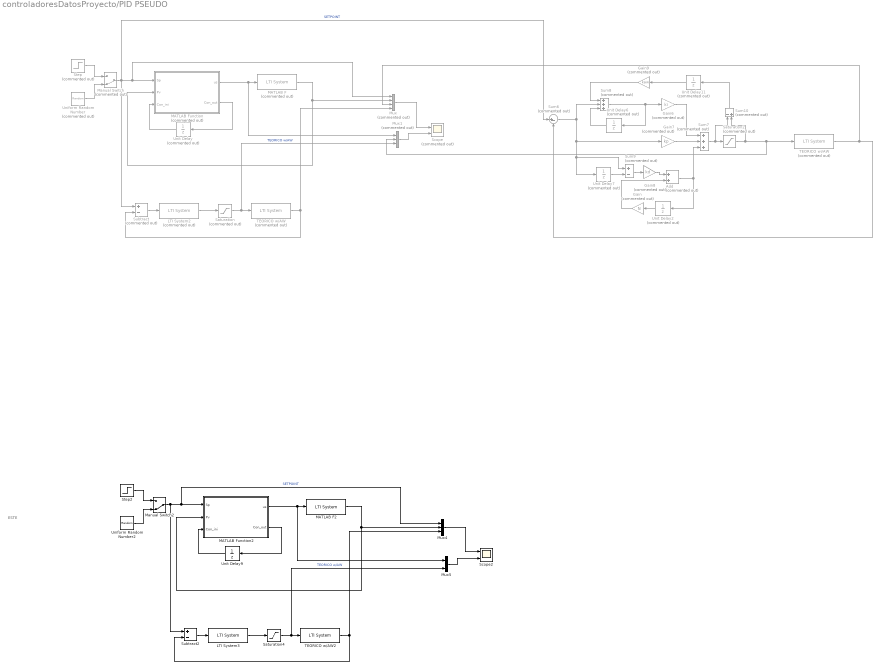
== system controladoresDatosProyecto/PID PSEUDO ==
  note: ESTE
  Add : Sum  Commented=on
  Gain : Gain  Commented=on  Gain=N
  Gain6 : Gain  Commented=on  Gain=ki
  Gain7 : Gain  Commented=on  Gain=kp
  Gain8 : Gain  Commented=on  Gain=kd
  Gain9 : Gain  Commented=on  Gain=kaw
  LTI System2 : cstblocks/LTI System  Commented=on  sys=Cz  IC=[]
  LTI System3 : cstblocks/LTI System  sys=Cpids  IC=[]
  MATLAB F : cstblocks/LTI System  Commented=on  sys=Gz  IC=[]
  MATLAB F2 : cstblocks/LTI System  sys=Gz  IC=[]
  MATLAB Function : MATLAB Function  Commented=on  TreatAsAtomicUnit=on
  MATLAB Function2 : MATLAB Function  TreatAsAtomicUnit=on
  Manual Switch : ManualSwitch  Commented=on  CurrentSetting=0
  Manual Switch2 : ManualSwitch  CurrentSetting=0
  Mux : Mux  Commented=on
  Mux1 : Mux  Commented=on  Inputs=3
  Mux4 : Mux  Inputs=3
  Mux5 : Mux  Inputs=2
  Saturation : Saturate  Commented=on  UpperLimit=100  LowerLimit=0
  Saturation2 : Saturate  Commented=on  UpperLimit=100  LowerLimit=0
  Saturation4 : Saturate  UpperLimit=100  LowerLimit=0
  Scope : Scope  Commented=on  NumInputPorts=2
  Scope2 : Scope  NumInputPorts=2
  Step : Step  Commented=on  Time=100  Before=18  After=15  SampleTime=0
  Step2 : Step  Time=100  Before=18  After=15  SampleTime=0
  Subtract : Sum  Commented=on  Inputs=+-
  Subtract2 : Sum  Inputs=+-
  Sum10 : Sum  Commented=on  Inputs=-+
  Sum6 : Sum  Commented=on  Inputs=|+-
  Sum7 : Sum  Commented=on  Inputs=+++
  Sum8 : Sum  Commented=on  Inputs=+++
  Sum9 : Sum  Commented=on  Inputs=+-
  TEORICO w/AW : cstblocks/LTI System  Commented=on  sys=Gz  IC=[]
  TEORICO w/AW2 : cstblocks/LTI System  sys=Gz  IC=[]
  TEORICO wi/AW : cstblocks/LTI System  Commented=on  sys=Gz  IC=[]
  Uniform Random Number : UniformRandomNumber  Commented=on  Minimum=0  Maximum=4.5  SampleTime=10
  Uniform Random Number2 : UniformRandomNumber  Minimum=0  Maximum=4.5  SampleTime=10
  Unit Delay : UnitDelay  Commented=on  InitialCondition=zeros(4,1)  SampleTime=Tm  HasFrameUpgradeWarning=on
  Unit Delay{2,6..7,11} (4 alike) : UnitDelay  Commented=on  SampleTime=Tm  HasFrameUpgradeWarning=on
  Unit Delay9 : UnitDelay  InitialCondition=zeros(4,1)  SampleTime=Tm  HasFrameUpgradeWarning=on
  wires:
  Unit Delay7/1 -> Sum9/2
  Unit Delay11/1 -> Gain9/1
  Unit Delay6/1 -> Sum8/3
  Unit Delay2/1 -> Gain/1
  TEORICO wi/AW/1 -> Sum6/2, Mux/3
  Gain9/1 -> Sum8/1
  Gain8/1 -> Add/1
  Sum9/1 -> Gain8/1
  Gain7/1 -> Sum7/2
  Add/1 -> Sum7/3, Unit Delay2/1
  Gain/1 -> Add/2
  TEORICO w/AW/1 -> Subtract/2, Mux/4
  MATLAB F/1 -> Mux/2, MATLAB Function/2(Pv)
  Sum10/1 -> Unit Delay11/1
  MATLAB Function/1(us) -> MATLAB F/1, Mux1/1
  Subtract/1 -> LTI System2/1
  Gain6/1 -> Sum7/1
  Step/1 -> Manual Switch/1
  Sum8/1 -> Unit Delay6/1, Gain6/1
  Sum7/1 -> Sum10/1, Saturation2/1
  MATLAB Function/2(Con_out) -> Unit Delay/1
  Mux/1 -> Scope/1
  Uniform Random Number/1 -> Manual Switch/2
  Saturation/1 -> TEORICO w/AW/1, Mux1/3  "TEORICO w/AW"
  Mux1/1 -> Scope/2
  Saturation2/1 -> TEORICO wi/AW/1, Mux1/2, Sum10/2
  LTI System2/1 -> Saturation/1
  Sum6/1 -> Sum9/1, Unit Delay7/1, Gain7/1, Sum8/2
  Unit Delay/1 -> MATLAB Function/3(Con_ini)
  Manual Switch/1 -> MATLAB Function/1(Sp), Mux/1, Sum6/1, Subtract/1  "SETPOINT"
  Step2/1 -> Manual Switch2/1
  Saturation4/1 -> Mux5/2, TEORICO w/AW2/1  "TEORICO w/AW"
  Mux5/1 -> Scope2/2
  Unit Delay9/1 -> MATLAB Function2/3(Con_ini)
  MATLAB F2/1 -> MATLAB Function2/2(Pv), Mux4/2
  LTI System3/1 -> Saturation4/1
  MATLAB Function2/1(us) -> Mux5/1, MATLAB F2/1
  TEORICO w/AW2/1 -> Mux4/3, Subtract2/2
  Subtract2/1 -> LTI System3/1
  Uniform Random Number2/1 -> Manual Switch2/2
  Manual Switch2/1 -> Subtract2/1, Mux4/1, MATLAB Function2/1(Sp)  "SETPOINT"
  Mux4/1 -> Scope2/1
  MATLAB Function2/2(Con_out) -> Unit Delay9/1

== matlab function controladoresDatosProyecto/BLOQUES CON F PROFE/MATLAB Function ==
  data: Sp input; u output; Pv input; Con_ini input; Con_out output
function [u,Con_out] = fcn(Sp,Pv,Con_ini)

en_1 = Con_ini(1);
en_2 = Con_ini(2);
u1_1 = Con_ini(3);
u1_2 = Con_ini(4);
Sp_1 = Con_ini(5);
u2_1 = Con_ini(6);

en = Sp - Pv;
u1 = 0.994677830358290*en - 1.874023294672252*en_1 + 0.955675954767192*en_2 + 1.246596963941606*u1_1 - 0.246596963941606*u1_2;
u2 = 0.010090239727970*Sp - 0.009890439594703*Sp_1 + 0.998001998667333*u2_1;
u = u1 + u2;

en_2 = en_1;
en_1 = en;
u1_2 = u1_1;
u1_1 = u1;
Sp_1 = Sp;
u2_1 = u2;

Con_out = [en_1; en_2; u1_1; u1_2; Sp_1; u2_1];

== matlab function controladoresDatosProyecto/PID IDEAL/MATLAB Function ==
  data: Sp input; us output; Pv input; Con_ini input; Con_out output
function [us, Con_out] = fcn(Sp, Pv, Con_ini)

en_1 = Con_ini(1);
I_error_1 = Con_ini(2);
difact = Con_ini(3);

umin = 0;
umax = 100;


kp = 26.4;
ki = 2.4;
kd = 137.9;

kaw = 0.1; 

en = Sp - Pv;
Ap = kp*en;
Ad = kd*(en-en_1);
I_error = en + I_error_1 + kaw*difact;
Ai = ki*I_error;
un = Ap + Ai + Ad;
us = un;

if un < umin 
    us = umin;
end
if un > umax 
    us = umax;
end

en_1 = en;
I_error_1 = I_error;
difact = us - un;
      
Con_out = [en_1; I_error_1; difact];

== matlab function controladoresDatosProyecto/PID PSEUDO/MATLAB Function ==
  data: Sp input; us output; Pv input; Con_ini input; Con_out output
% function [us, Con_out] = fcn(Sp, Pv, Con_ini)
% 
% en_1 = Con_ini(1);
% en_2 = Con_ini(2);
% un_1 = Con_ini(3);
% un_2 = Con_ini(4);
% difact = Con_ini(5);
% umin = 0;
% umax = 100;
% kaw = 1; 
% 
% en = Sp - Pv;
% un = 11.554000000000000*en - 21.536656000000001*en_1 + 10.035804400000000*en_2 + 1.966200000000000*un_1 - 0.966200000000000*un_2+ kaw*difact;
% 
% us = un;
% 
% if un < umin 
%     us = umin;
% end
% if un > umax 
%     us = umax;
% end
% 
% en_2 = en_1;
% en_1 = en;
% un_2 = un_1;
% un_1 = un;
% difact = us - un;
%          
% Con_out = [en_1; en_2; un_1; un_2; difact];



function [us, Con_out] = fcn(Sp, Pv, Con_ini)

en_1 = Con_ini(1);
I_error_1 = Con_ini(2);
difact = Con_ini(3);
Ad_1 = Con_ini(4);

umin = 0;
umax = 100;

kp =     -1.604800882321478;
ki =    1.572437869822466;
kd =    11.586363012499012;
kaw=0; 
N = 0.9662;


en = Sp - Pv;
Ap = kp*en;
Ad = kd*(en-en_1) + N*Ad_1;
I_error = en + I_error_1 + kaw*difact;
Ai = ki*I_error;
un = Ap + Ai + Ad;
us = un;

if un < umin 
    us = umin;
end
if un > umax 
    us = umax;
end

en_1 = en;
I_error_1 = I_error;
difact = us - un;
Ad_1 = Ad;
      
Con_out = [en_1; I_error_1; difact; Ad_1];

== matlab function controladoresDatosProyecto/PID IDEAL/MATLAB Function1 ==
  data: Sp input; us output; Pv input; Con_ini input; Con_out output
function [us, Con_out] = fcn(Sp, Pv, Con_ini)

en_1 = Con_ini(1);
I_error_1 = Con_ini(2);
difact = Con_ini(3);

umin = 0;
umax = 100;

% 1 SEGUNDOS
Kp = 6.629839917619998;
Ki = 2.333050066190001;
Kd = 0.927610016190000;

% 2 SEGUNDOS
% Kp= 9.396787156500000;
% Ki = 1.683836421750000;
% Kd = 12.144376421750001;

kaw = 0.1; 

en = Sp - Pv;
Ap = Kp*en;
Ad = Kd*(en-en_1);
I_error = en + I_error_1 + kaw*difact;
Ai = Ki*I_error;
un = Ap + Ai + Ad;
us = un;

if un < umin 
    us = umin;
end
if un > umax 
    us = umax;
end

en_1 = en;
I_error_1 = I_error;
difact = us - un;
      
Con_out = [en_1; I_error_1; difact];

== matlab function controladoresDatosProyecto/PI-D/MATLAB Function1 ==
  data: Sp input; us output; Pv input; Con_ini input; Con_out output
function [us, Con_out] = fcn(Sp, Pv, Con_ini)

yn_1 = Con_ini(1);
I_error_1 = Con_ini(2);
dif_act = Con_ini(3);

umin = 0;
umax = 100;

%1 SEGUNDOS
% Kp = 11.143200000000000;
% Ki = 2.785800000000000;
% Kd =1;
% Ka= 0.1; 

%2 SEGUNDOS
Kp = 23.243727600000000;
Ki = 2.352272400000000;
Kd =1;
Ka= 0.1; 


en = Sp - Pv;
A_p = Kp * en;
A_d = Kd * (Pv-yn_1);
I_error = en + I_error_1 + Ka*dif_act;  
A_i = Ki* I_error;
Uc = A_p + A_i - A_d;
us = Uc;

if Uc < umin 
    us = umin;
end
if Uc > umax 
    us = umax;
end

yn_1 = Pv;
I_error_1 = I_error;
dif_act = us - Uc;
      
Con_out = [yn_1; I_error_1; dif_act];

== matlab function controladoresDatosProyecto/PID PSEUDO/MATLAB Function2 ==
  data: Sp input; us output; Pv input; Con_ini input; Con_out output
% function [us, Con_out] = fcn(Sp, Pv, Con_ini)
% 
% en_1 = Con_ini(1);
% en_2 = Con_ini(2);
% un_1 = Con_ini(3);
% un_2 = Con_ini(4);
% difact = Con_ini(5);
% umin = 0;
% umax = 100;
% kaw = 1; 
% 
% en = Sp - Pv;
% un = 11.554000000000000*en - 21.536656000000001*en_1 + 10.035804400000000*en_2 + 1.966200000000000*un_1 - 0.966200000000000*un_2+ kaw*difact;
% 
% us = un;
% 
% if un < umin 
%     us = umin;
% end
% if un > umax 
%     us = umax;
% end
% 
% en_2 = en_1;
% en_1 = en;
% un_2 = un_1;
% un_1 = un;
% difact = us - un;
%          
% Con_out = [en_1; en_2; un_1; un_2; difact];



function [us, Con_out] = fcn(Sp, Pv, Con_ini)

en_1 = Con_ini(1);
I_error_1 = Con_ini(2);
difact = Con_ini(3);
Ad_1 = Con_ini(4);

umin = 0;
umax = 100;

% 1 SEGUNDOS
% Kp = 6.107123008000580;
% Ki = 2.786107391999990;
% Kd = 4.250769599999430;
% kaw=0.1; 
% N = 0.98;

% 2 SEGUNDOS
Kp = 21.746325533681762;
Ki = 2.108194038461562;
Kd = -1.640519572143324;
N = 0.9662;
kaw=0.1; 


en = Sp - Pv;
Ap = Kp*en;
Ad = Kd*(en-en_1) + N*Ad_1;
I_error = en + I_error_1 + kaw*difact;
Ai = Ki*I_error;
un = Ap + Ai + Ad;
us = un;

if un < umin 
    us = umin;
end
if un > umax 
    us = umax;
end

en_1 = en;
I_error_1 = I_error;
difact = us - un;
Ad_1 = Ad;
      
Con_out = [en_1; I_error_1; difact; Ad_1];

== matlab function controladoresDatosProyecto/PI-PD PSEUDO/MATLAB Function3 ==
  data: Sp input; us output; Pv input; Con_ini input; Con_out output
function [us, Con_out] = fcn(Sp, Pv, Con_ini)

yn_1 = Con_ini(1);
I_error_1 = Con_ini(2);
dif_act = Con_ini(3);
Ad_1 = Con_ini(4);

umin = 0;
umax = 100;

Kpi = 4.328000000000000;
Kpd = 0.557916666666666;
Ki = 2.246000000000000;
Kd = 0.002643333333334;
N = 0.904;
Ka= 0.1; 

en =  Sp - Pv;
A_p = Kpi * en;
I_error = en + I_error_1 + Ka*dif_act;    
A_i = Ki* I_error;
U1 = A_p + A_i;

A_p1 = Kpd * Pv;
A_d1 = Kd * (Pv - yn_1) + N*Ad_1;
U2 = A_p1 + A_d1;

Uc = U1 - U2;
us = Uc;


if Uc < umin 
    us = umin;
end
if Uc > umax 
    us = umax;
end

yn_1 = Pv;
I_error_1 = I_error;
dif_act = us - Uc;
Ad_1 = A_d1;
      
Con_out = [yn_1; I_error_1; dif_act; Ad_1];

== matlab function controladoresDatosProyecto/PI-PD/MATLAB Function3 ==
  data: Sp input; us output; Pv input; Con_ini input; Con_out output
function [us, Con_out] = fcn(Sp, Pv, Con_ini)

yn_1 = Con_ini(1);
I_error_1 = Con_ini(2);
difact = Con_ini(3);


umin = 0;
umax = 100;


kp1 = 8.223313200000000;
ki = 2.572686800000000;
kd = 0.568600000000000;
kp2 = 0.431400000000000;
kaw = 0.01; 

en = Sp - Pv;
Ap1 = kp1*en;
I_error = en + I_error_1 + kaw*difact;
Ai = ki*I_error;
u1 = Ap1 + Ai;

Ap2 = kp2*Pv;
Ad = kd*(Pv-yn_1);
u2 = Ap1 + Ad;
un = u1 - u2;
us = un;

if un < umin 
    us = umin;
end
if un > umax 
    us = umax;
end

yn_1 = Pv;
I_error_1 = I_error;
difact = us - un;
      
Con_out = [yn_1; I_error_1; difact;];

== matlab function controladoresDatosProyecto/PARCIAL/UPI-D ==
  data: Sp input; us output; Pv input; Con_ini input; Con_out output
function [us, Con_out] = fcn(Sp, Pv, Con_ini)

yn_1 = Con_ini(1);
I_error_1 = Con_ini(2);

umin = 0;
umax = 20;


Kp = 0.164521719000000;
Ki = 0.024388281000000;
Kd =4.593300000000000e-05;


en = Sp - Pv;
A_p = Kp * en;
A_d = Kd * (Pv-yn_1);
I_error = en + I_error_1;  
A_i = Ki* I_error;
Uc = A_p + A_i - A_d;
us = Uc;

if Uc < umin 
    us = umin;
end
if Uc > umax 
    us = umax;
end

yn_1 = Pv;
I_error_1 = I_error;
      
Con_out = [yn_1; I_error_1];

== matlab function controladoresDatosProyecto/PARCIAL/UCASCADA ==
  data: Sp input; u2 output; Pv input; Pv1 input; Con_ini input; Con_out output
function [u2,Con_out] = fcn(Sp,Pv,Pv1,Con_ini)

en_1 = Con_ini(1);
u1_1 = Con_ini(2);
en2_1 = Con_ini(3);
en2_2 = Con_ini(4);
u2_1 = Con_ini(5);
u2_2 = Con_ini(6);

en = Sp - Pv;
u1 = 0.728387630774072*en - 0.713265246774072*en_1+1*u1_1;
en_1 = en;
u1_1 = u1;

en2 = u1 - Pv1;
u2 = 0.207403060303267*en2 - 0.360891769937693*en2_1 + 0.187564737267579*en2_2 + 1.670320046035639*u2_1 - 0.670320046035639*u2_2;
en2_2 = en2_1;
en2_1 = en2;
u2_2 = u2_1;
u2_1 = u2;

Con_out = [en_1; u1_1; en2_1; en2_2; u2_1; u2_2];

== matlab function controladoresDatosProyecto/CASCADA PROFE/MATLAB Function1 ==
  data: Sp input; u2 output; Pv input; Pv1 input; Con_ini input; Con_out output
function [u2,Con_out] = fcn(Sp,Pv,Pv1,Con_ini)

en_1 = Con_ini(1);
u1_1 = Con_ini(2);
en2_1 = Con_ini(3);
en2_2 = Con_ini(4);
u2_1 = Con_ini(5);
u2_2 = Con_ini(6);

en = Sp - Pv;
u1 = 0.403367728657773*en - 0.397984326537773*en_1  + 1*u1_1;
% + 0.972388366801247*u1_1;
en_1 = en;
u1_1 = u1;

en2 = u1 - Pv1;
u2 = 0.117993268371376*en2 - 0.206313032319716*en2_1 + 0.106792486736058*en2_2 + 1.670320046035639*u2_1 - 0.670320046035639*u2_2;
en2_2 = en2_1;
en2_1 = en2;
u2_2 = u2_1;
u2_1 = u2;

Con_out = [en_1; u1_1; en2_1; en2_2; u2_1; u2_2];

== matlab function controladoresDatosProyecto/PI-D/MATLAB Function ==
  data: Sp input; us output; Pv input; Con_ini input; Con_out output
function [us, Con_out] = fcn(Sp, Pv, Con_ini)

yn_1 = Con_ini(1);
I_error_1 = Con_ini(2);
difact = Con_ini(3);

umin = 0;
umax = 100;


kp = 66.17;
ki = 1;
kd = 200;

kaw = 1/(ki*kd); 

en = Sp - Pv;
Ap = kp*en;
Ad = kd*(Pv-yn_1);
I_error = en + I_error_1 + kaw*difact;
Ai = ki*I_error;
un = Ap + Ai - Ad;
us = un;

if un < umin 
    us = umin;
end
if un > umax 
    us = umax;
end

yn_1 = Pv;
I_error_1 = I_error;
difact = us - un;
      
Con_out = [yn_1; I_error_1; difact];

== matlab function controladoresDatosProyecto/I-PD/MATLAB Function ==
  data: Sp input; us output; Pv input; Con_ini input; Con_out output
function [us, Con_out] = fcn(Sp, Pv, Con_ini)

yn_1 = Con_ini(1);
I_error_1 = Con_ini(2);
difact = Con_ini(3);

umin = 0;
umax = 100;

%1 SEGUNDO
% kp = 2.512097499999999;
% ki = 1.978400000000000;
% kd = 11.162902500000001;
% kaw = 0.1; 

%2 SEGUNDO
kp = 54.036070000000002;
ki = 5;
kd = 63.663930000000001;
kaw = 0.1; 

en = Sp - Pv;
Ap = kp*Pv;
Ad = kd*(Pv-yn_1);
I_error = en + I_error_1 + kaw*difact;
Ai = ki*I_error;
un = -Ap + Ai - Ad;
us = un;

if un < umin 
    us = umin;
end
if un > umax 
    us = umax;
end

yn_1 = Pv;
I_error_1 = I_error;
difact = us - un;
      
Con_out = [yn_1; I_error_1; difact];

== matlab function controladoresDatosProyecto/PID IDEAL ECUACIONES/MATLAB Function ==
  data: Sp input; us output; Pv input; Con_ini input; Con_out output
function [us, Con_out] = fcn(Sp, Pv, Con_ini)
 
en_1 = Con_ini(1);
en_2 = Con_ini(2);
un_1 = Con_ini(3);
difact = Con_ini(4);
umin = 0;
umax = 100;
kaw = 0.1; 
 
en = Sp - Pv;
un = 166.71*en - 302.24523*en_1 + 137.86917*en_2 + 1*un_1 + kaw*difact;
 
us = un;
 
if un < umin 
    us = umin;
end
if un > umax 
    us = umax;
end
 
en_2 = en_1;
en_1 = en;
un_1 = un;
difact = us - un;
         
Con_out = [en_1; en_2; un_1; difact];

== matlab function controladoresDatosProyecto/PI-PD/MATLAB Function ==
  data: Sp input; us output; Pv input; Con_ini input; Con_out output
function [us, Con_out] = fcn(Sp, Pv, Con_ini)

yn_1 = Con_ini(1);
I_error_1 = Con_ini(2);
difact = Con_ini(3);


umin = 0;
umax = 100;


kp1 = 72.3700;
ki = 1.1000;
kd = 58.1800;
kp2 = 0.8800;

kaw = 0.1; 

en = Sp - Pv;
Ap1 = kp1*en;
I_error = en + I_error_1 + kaw*difact;
Ai = ki*I_error;
u1 = Ap1 + Ai;

Ap2 = kp2*Pv;
Ad = kd*(Pv-yn_1);
u2 = Ap1 + Ad;
un = u1 - u2;
us = un;

if un < umin 
    us = umin;
end
if un > umax 
    us = umax;
end

yn_1 = Pv;
I_error_1 = I_error;
difact = us - un;
      
Con_out = [yn_1; I_error_1; difact;];

== matlab function controladoresDatosProyecto/PI-PD ECUACIONES/MATLAB Function ==
  data: Sp input; us output; Pv input; Con_ini input; Con_out output
function [us, Con_out] = fcn(Sp, Pv, Con_ini)
 
en_1 = Con_ini(1);
Pv_1 = Con_ini(2);
un_1 = Con_ini(3);
difact = Con_ini(4);


umin = 0;
umax = 100;
kaw = 0.1; 
 %CPI
en = Sp - Pv;
un = 73.469999999999999*en - 72.370000000000005*en_1 + 1*un_1 + kaw*difact;
 %CPD
 u2n = 59.060000000000002*Pv - 58.180000000000000*Pv_1;

 unt = un - u2n;
us = unt;
 
if unt < umin 
    us = umin;
end
if unt > umax 
    us = umax;
end
 
Pv_1 = Pv;
en_1 = en;
un_1 = un;
difact = us - un;
         
Con_out = [en_1; Pv_1; un_1; difact];

== matlab function controladoresDatosProyecto/CASCADA/MATLAB Function ==
  data: Sp input; Usat_pwm output; Pv_vout input; Pv_W input; Con_ini input; Con_out output
function [Usat_pwm, Con_out] = fcn(Sp, Pv_vout,Pv_W, Con_ini)
En1_1 = Con_ini(1);
En1_2 = Con_ini(2);
U_velocidad_1  = Con_ini(3);
U_velocidad_2 = Con_ini(4);
En2_1 = Con_ini(5);
En2_2 = Con_ini(6);
U_pwm_1 = Con_ini(7);
U_pwm_2 = Con_ini(8);
Umax = 8100;

En1 = Sp - Pv_vout;
U_velocidad =3.12*En1 - 5.928*En1_1 + 2.896*En1_2 + 1.59*U_velocidad_1 -0.59*U_velocidad_2;

Usat_velocidad = U_velocidad;

if U_velocidad < 0
    Usat_velocidad = 0;
end
if U_velocidad > Umax
    Usat_velocidad = Umax;
end

En2 = Usat_velocidad-Pv_W;
U_pwm = 0.0032*En2 - 0.00064*En2_1 + 0.002624*En2_2 + 1.565*U_pwm_1 - 0.565*U_pwm_2;
Usat_pwm = U_pwm;

if U_pwm < 0
    Usat_pwm= 0;
end
if U_pwm > 100
    Usat_pwm = 100;
end


 En1_2 = En1_1;
 En1_1 = En1;

 U_velocidad_2 = U_velocidad_1; 
 U_velocidad_1 = U_velocidad;

 U_pwm_2 = U_pwm_1; 
 U_pwm_1 = U_pwm;

Con_out = [En1_1; En1_2; U_velocidad_1; U_velocidad_2;U_pwm_1;U_pwm_2; En2_1;En2_2;];

== matlab function controladoresDatosProyecto/PI-PD2/MATLAB Function ==
  data: Sp input; us output; Pv input; Con_ini input; Con_out output
function [us, Con_out] = fcn(Sp, Pv, Con_ini)
 yn_1 = Con_ini(1);
I_error_1 = Con_ini(2);
difact = Con_ini(3);
Ad_1 = Con_ini(4);


umin = 0;
umax = 100;

kp1 = 0.497600000000000;
kp2 = 3.366696997270255;
ki =0.105500000000000;
kd = 15.803303002729747;
N = 0.6703;

kaw = 0.1; 

en = Sp - Pv;
Ap1 = kp1*en;
I_error = en + I_error_1 + kaw*difact;
Ai = ki*I_error;
u1 = Ap1 + Ai;

Ap2 = kp2*Pv;
Ad = kd*(Pv-yn_1) + N*Ad_1;
u2 = Ap2 + Ad;

un = u1 - u2;
us = un;

if un < umin 
    us = umin;
end
if un > umax 
    us = umax;
end

yn_1 = Pv;
I_error_1 = I_error;
difact = us - un;
Ad_1=Ad;

Con_out = [yn_1; I_error_1; Ad_1; difact];
